simulink model "button_to_led"  (R2016a)
settings: Solver=FixedStepDiscrete  StartTime=0.0  StopTime=500000  FixedStep=1  RelTol=1e-3
libraries: hdlsllib x2, simulink x1
settings Model: Creator=duyvu  LastModifiedBy=duyvu

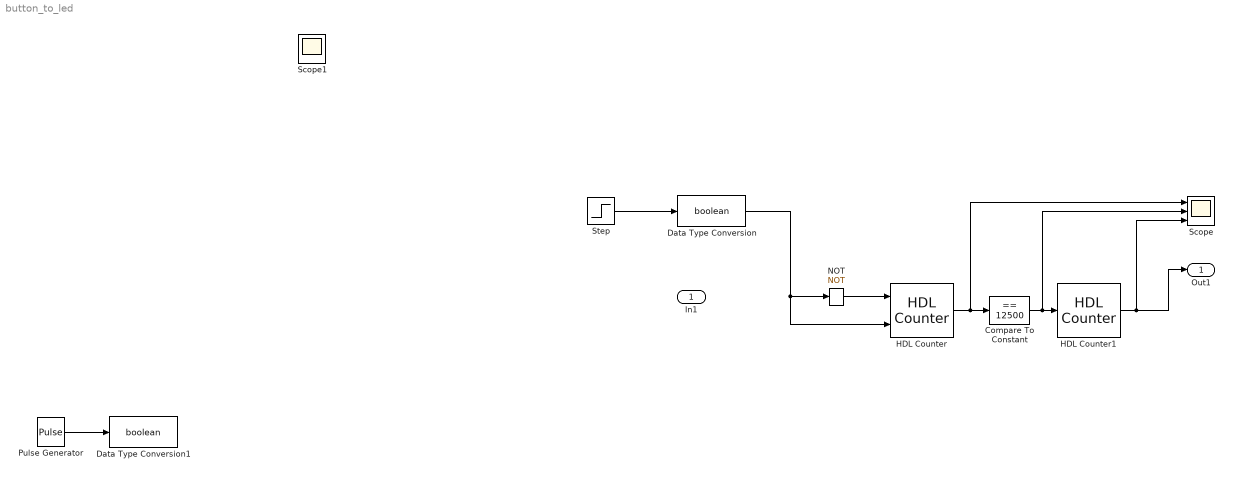
== system button_to_led ==
  In1 : Inport
  Compare To Constant : simulink/Logic and Bit Operations/Compare To Constant  relop===  const=12500  OutDataTypeStr=boolean
  Data Type Conversion : DataTypeConversion  OutDataTypeStr=boolean
  Data Type Conversion1 : DataTypeConversion  OutDataTypeStr=boolean
  HDL Counter : hdlsllib/HDL Operations/HDL Counter  CountType=Count limited  CountInit=0  CountStep=1  CountMax=50000  CountFromType=Initial value  CountFrom=0  CountResetPort=on  CountLoadPort=off  CountEnbPort=on  CountDirPort=off  CountDataType=Unsigned  CountWordLen=32  CountFracLen=0  CountSampTime=1
  HDL Counter1 : hdlsllib/HDL Operations/HDL Counter  CountType=Free running  CountInit=0  CountStep=1  CountMax=25  CountFromType=Initial value  CountFrom=0  CountResetPort=off  CountLoadPort=off  CountEnbPort=on  CountDirPort=off  CountDataType=Unsigned  CountWordLen=1  CountFracLen=0  CountSampTime=1
  NOT : Logic  Operator=NOT  IconShape=distinctive  AllPortsSameDT=off  OutDataTypeStr=boolean
  Pulse Generator : DiscretePulseGenerator  Period=25000  PulseWidth=5
  Scope : Scope  NumInputPorts=3
  Scope1 : Scope
  Step : Step  Time=25000  SampleTime=1
  Out1 : Outport
  wires:
  HDL Counter/1 -> Scope/1, Compare To Constant/1
  Compare To Constant/1 -> HDL Counter1/1, Scope/2
  HDL Counter1/1 -> Scope/3, Out1/1
  Step/1 -> Data Type Conversion/1
  NOT/1 -> HDL Counter/1
  Pulse Generator/1 -> Data Type Conversion1/1
  Data Type Conversion/1 -> NOT/1, HDL Counter/2
